simulink library "Lib_VehicleModel"  (R2019b)
settings: Solver=VariableStepAuto  StartTime=0.0  StopTime=10.0  RelTol=1e-3
settings Model: Creator=esterle  LastModifiedBy=kessler
settings DataIOCC: ReturnWorkspaceOutputs=off
settings DebuggingCC: ArithmeticOperatorsInVariantConditions=warning
settings SFSimCC: SimUseLocalCustomCode=off  CustomCodeUndefinedFunction=UseInterfaceOnly
settings RTWCC: RTWUseLocalCustomCode=off

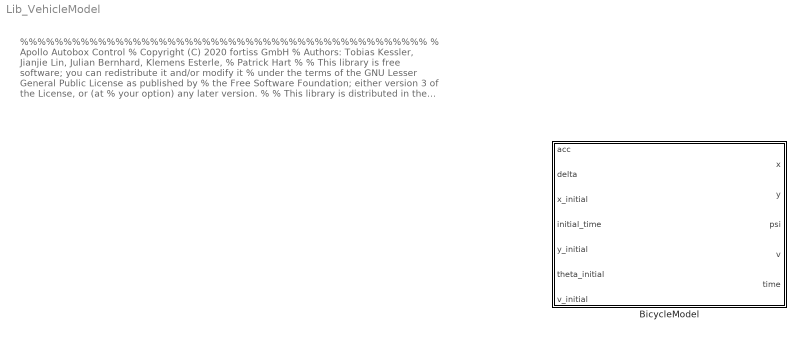
== system Lib_VehicleModel ==
  note: %%%%%%%%%%%%%%%%%%%%%%%%%%%%%%%%%%%%%%%%%%%%%%%
      | % Apollo Autobox Control
      | % Copyright (C) 2020 fortiss GmbH
      | % Authors: Tobias Kessler, Jianjie Lin, Julian Bernhard, Klemens Esterle,
      | % Patrick Hart
      | %
      | % This library is free software; you can redistribute it and/or modify it
      | % under the terms of the GNU Lesser General Public License as published by
      | % the Free Software Foundation; either version 3 of the License, or (at
      | % your option) any later version.
      | %
      | % This library is distributed in the hope that it will be useful, but
      | % WITHOUT ANY WARRANTY; without even the implied warranty of
      | % MERCHANTABILITY or FITNESS FOR A PARTICULAR PURPOSE. See the GNU Lesser
      | % General Public License for more details.
      | %
      | % You should have received a copy of the GNU Lesser General Public License
      | % along with this library; if not, write to the Free Software Foundation,
      | % Inc., 51 Franklin Street, Fifth Floor, Boston, MA 02110-1301, USA.
      | %%%%%%%%%%%%%%%%%%%%%%%%%%%%%%%%%%%%%%%%%%%%%%%
  BicycleModel : Subsystem  mask{l=2.6}
      mask prompts: l "VehicleLength"
      mask DialogControl DescGroupVar Prompt: Parameters Vehicle Model

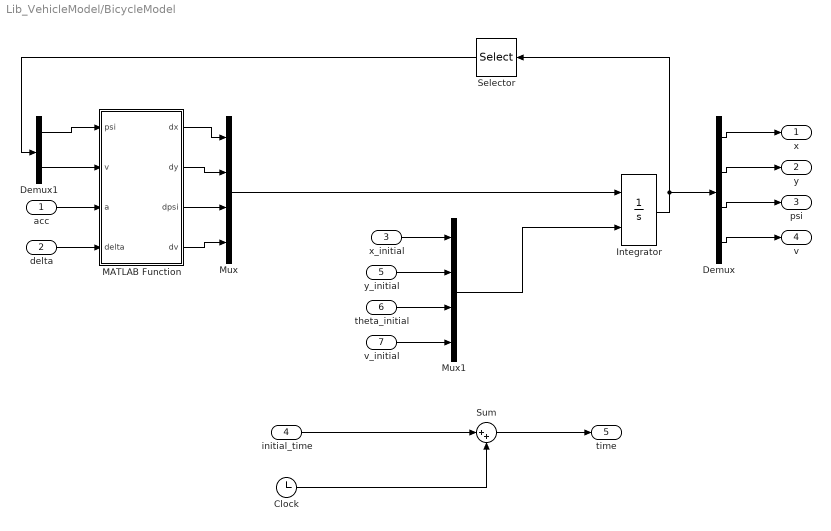
== system Lib_VehicleModel/BicycleModel ==
  acc : Inport
  delta : Inport  Port=2
  "x_initial " : Inport  Port=3
  initial_time : Inport  Port=4
  y_initial : Inport  Port=5
  theta_initial : Inport  Port=6
  v_initial : Inport  Port=7
  Clock : Clock
  Demux : Demux
  Demux1 : Demux  Outputs=2
  Integrator : Integrator  InitialConditionSource=external  InitialCondition=[0 0 0 1]
  MATLAB Function : MATLAB Function  TreatAsAtomicUnit=on
  Mux : Mux
  Mux1 : Mux
  Selector : Selector  InputPortWidth=4  IndexOptions=Index vector (dialog)  Indices=[3 4]  OutputSizes=1
  Sum : Sum  Inputs=|++
  x : Outport  VectorParamsAs1DForOutWhenUnconnected=off
  y : Outport  Port=2  VectorParamsAs1DForOutWhenUnconnected=off
  psi : Outport  Port=3  VectorParamsAs1DForOutWhenUnconnected=off
  v : Outport  Port=4  VectorParamsAs1DForOutWhenUnconnected=off
  time : Outport  Port=5  VectorParamsAs1DForOutWhenUnconnected=off
  wires:
  Clock/1 -> Sum/2
  initial_time/1 -> Sum/1
  v_initial/1 -> Mux1/4
  theta_initial/1 -> Mux1/3
  y_initial/1 -> Mux1/2
  "x_initial "/1 -> Mux1/1
  Mux1/1 -> Integrator/2
  Sum/1 -> time/1
  MATLAB Function/1(dx) -> Mux/1
  Demux/1 -> x/1
  MATLAB Function/3(dpsi) -> Mux/3
  Demux/2 -> y/1
  MATLAB Function/2(dy) -> Mux/2
  Mux/1 -> Integrator/1
  Demux/3 -> psi/1
  delta/1 -> MATLAB Function/4(delta)
  acc/1 -> MATLAB Function/3(a)
  Demux/4 -> v/1
  Integrator/1 -> Selector/1, Demux/1
  MATLAB Function/4(dv) -> Mux/4
  Selector/1 -> Demux1/1
  Demux1/2 -> MATLAB Function/2(v)
  Demux1/1 -> MATLAB Function/1(psi)

== matlab function Lib_VehicleModel/BicycleModel/MATLAB Function ==
  data: psi input; dx output; v input; a input; delta input; dy output; dpsi output; dv output; l parameter
function [dx ,dy, dpsi, dv] = fcn(psi, v, a, delta, l)

% calculate state derivatives
dx = v * cos(psi);
dy = v * sin(psi);
dpsi = v * tan(delta)/l;
dv = a;
